simulink model "Vehicle_Model_14DOF"  (R2020a)
settings: Solver=ode23s  StartTime=0.0  StopTime=8  RelTol=1e-2  EnableMultiTasking=on
model workspace (MAT data in the model file):
  Csfl = 100
  Csfr = 100
  Csrl = 100
  Csrr = 100
  Hp = 0.35
  Ksfl = 100
  Ksfr = 100
  Ksrl = 100
  Ksrr = 100
undefined symbols (not defined in the file): sigbuilder_block
libraries: simulink_extras x6, simulink x1
(part 1 of 3)
settings Model: Creator=Admin  LastModifiedBy=Asser Roshdy
settings SolverCC: ZeroCrossControl=DisableAll
settings DataIOCC: ReturnWorkspaceOutputs=off
settings OptimizationCC: LifeSpan=inf
settings DebuggingCC: AllowSymbolicDim=off  StateNameClashWarn=warning  ArithmeticOperatorsInVariantConditions=warning
settings HardwareCC: ProdBitPerSizeT=32  ProdBitPerPtrDiffT=32  ProdWordSize=32  ProdHWDeviceType=Specified
settings SFSimCC: SimUseLocalCustomCode=off  CustomCodeUndefinedFunction=UseInterfaceOnly
settings RTWCC: RTWUseLocalCustomCode=off
settings CodeAppCC: StateflowObjectComments=on
settings SimscapeCC: SimscapeNormalizeSystem=off
settings ConfigurationSet: Description=SimMechanics 2G

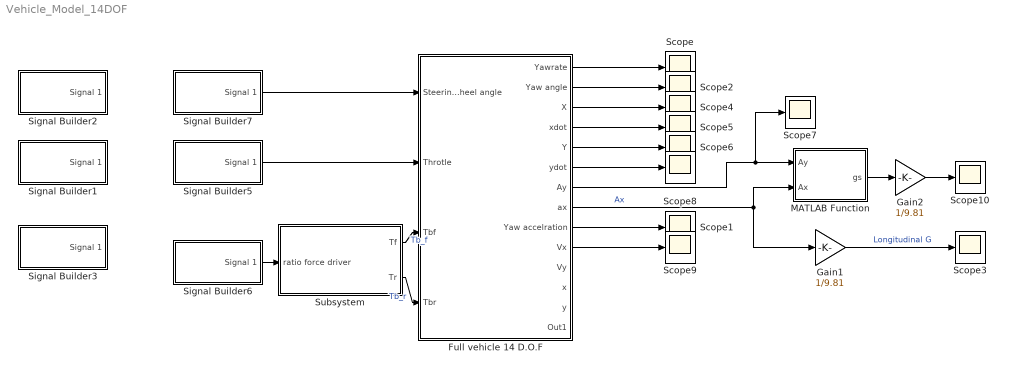
== system Vehicle_Model_14DOF ==
  "Full vehicle 14 D.O.F " : Subsystem  mask{P_A=0.75, Ms=240, Mufr=11.5, Mufl=11.5, Murr=13, Murl=13, wf=1.195, wr=1.180, b=0.753, a=0.826, H=0.314, Hr=0.060, Hp=0.096, Ip=38, Ir=146, Izz=125, Ksrr=16000, Ksrl=16000, Ksfr=21000, Ksfl=21000, Cdfr=781, Cdfl=781, Cdrr=944, Cdrl=944, Ktfr=120000, Ktfl=120000, Ktrr=120000, Ktrl=120000, Iwf=0.36, Iwr=0.36, Rw=0.260, R1=19.91, R2=13.86, R3=10.61, R4=8.535, Ro=1.18, Cd=0.91, Ar=1.2, Cl=2.1}
      mask prompts: P_A "Percentage Ackerman"; Ms "Sprung mass"; Mufr "Unsprung mass front right"; Mufl "Unsprung mass front left"; Murr "Unsprunf mass rear right"; Murl "Unsprunf mass rear left"; wf "Track width front"; wr "Track width rear"; b "C.G distance from the rear axle"; a "C.G distance from the front axle"; H "CG height"; Hr "Roll center height"; Hp "pitch center height"; Ip "Ixx"; Ir "Iyy"; Ksrr "Rear right susspension spring stiffness"; Ksrl "Rear left susspension spring stiffness"; Ksfr "Front right susspension spring stiffness"; Ksfl "Front left susspension spring stiffness"; Cdfr "Damping coefcient front right"; Cdfl "Damping coefcient front left"; Cdrr "Damping coefcient rear right"; Cdrl "Damping coefcient rear right"; Ktfr "Tire stiffness front right"; Ktfl "Tire stiffness front left"; Ktrr "Tire stiffness rear right"; Ktrl "Tire stiffness rear left"; Iwf "Tire inertia front"; Iwr "Tire inertia rear"; Rw "Tire rolling radius"; R1 "reduction 1"; R2 "reduction 2"; R3 "reduction 3"; R4 "reduction 4"; Ro "Air density"; Cd "Coefficient of drag"; Ar "Frontal area"; Cl "Coffiecient of downforce"
  Gain1 : Gain  Gain=1/9.81
  Gain2 : Gain  Gain=1/9.81
  MATLAB Function : MATLAB Function  TreatAsAtomicUnit=on
  Scope{,1..10} (11 alike) : Scope
  Signal Builder1 : Subsystem  Tag=STV Subsys  LoadFcn=sigbuilder_block('load');  StartFcn=sigbuilder_block('start');  StopFcn=sigbuilder_block('stop');  ClipboardFcn=sigbuilder_block('clipboard');  mask(Sigbuilder block){tuvar=[0:10]}
      mask help: Simulink:masks:SigbuilderBlock_MD
      mask init:
      | if ~strcmp(get_param(bdroot(gcbh),'SimulationStatus'),'stopped') tuvar = sigbuilder_block('maskInit'); end
      settings: CopyFcn=sigbuilder_block('copy');  DeleteFcn=sigbuilder_block('delete');  ModelCloseFcn=sigbuilder_block('modelClose');  PreSaveFcn=sigbuilder_block('preSave');  PauseFcn=sigbuilder_block('pause');  ContinueFcn=sigbuilder_block('continue');  NameChangeFcn=sigbuilder_block('namechange');  OpenFcn=sigbuilder_block('open',[84 117 1141.5 490.5 ]);  CloseFcn=sigbuilder_block('close');
      mask Display: plot(0, 0, 100, 100,[2, 2, 32, 32, 2], [68, 8, 8, 68, 68],[32, 2], [38, 38], [32, 19, 2],[53, 60, 44], [32, 17, 17, 2],[16, 16, 31, 31]);txt = getActiveGroup(gcbh);text(2, 100, txt,'verticalAlignment', 'top');
  Signal Builder2 : Subsystem  Tag=STV Subsys  LoadFcn=sigbuilder_block('load');  StartFcn=sigbuilder_block('start');  StopFcn=sigbuilder_block('stop');  ClipboardFcn=sigbuilder_block('clipboard');  mask(Sigbuilder block){tuvar=[0:10]}
      mask help: Simulink:masks:SigbuilderBlock_MD
      mask init:
      | if ~strcmp(get_param(bdroot(gcbh),'SimulationStatus'),'stopped') tuvar = sigbuilder_block('maskInit'); end
      settings: CopyFcn=sigbuilder_block('copy');  DeleteFcn=sigbuilder_block('delete');  ModelCloseFcn=sigbuilder_block('modelClose');  PreSaveFcn=sigbuilder_block('preSave');  PauseFcn=sigbuilder_block('pause');  ContinueFcn=sigbuilder_block('continue');  NameChangeFcn=sigbuilder_block('namechange');  OpenFcn=sigbuilder_block('open',[6 30 1428 681.75 ]);  CloseFcn=sigbuilder_block('close');
      mask Display: plot(0, 0, 100, 100,[2, 2, 32, 32, 2], [68, 8, 8, 68, 68],[32, 2], [38, 38], [32, 19, 2],[53, 60, 44], [32, 17, 17, 2],[16, 16, 31, 31]);txt = getActiveGroup(gcbh);text(2, 100, txt,'verticalAlignment', 'top');
  Signal Builder3 : Subsystem  Tag=STV Subsys  LoadFcn=sigbuilder_block('load');  StartFcn=sigbuilder_block('start');  StopFcn=sigbuilder_block('stop');  ClipboardFcn=sigbuilder_block('clipboard');  mask(Sigbuilder block){tuvar=[0:10]}
      mask help: Simulink:masks:SigbuilderBlock_MD
      mask init:
      | if ~strcmp(get_param(bdroot(gcbh),'SimulationStatus'),'stopped') tuvar = sigbuilder_block('maskInit'); end
      settings: CopyFcn=sigbuilder_block('copy');  DeleteFcn=sigbuilder_block('delete');  ModelCloseFcn=sigbuilder_block('modelClose');  PreSaveFcn=sigbuilder_block('preSave');  PauseFcn=sigbuilder_block('pause');  ContinueFcn=sigbuilder_block('continue');  NameChangeFcn=sigbuilder_block('namechange');  OpenFcn=sigbuilder_block('open',[20.25 37.5 1030.5 470.25 ]);  CloseFcn=sigbuilder_block('close');
      mask Display: plot(0, 0, 100, 100,[2, 2, 32, 32, 2], [68, 8, 8, 68, 68],[32, 2], [38, 38], [32, 19, 2],[53, 60, 44], [32, 17, 17, 2],[16, 16, 31, 31]);txt = getActiveGroup(gcbh);text(2, 100, txt,'verticalAlignment', 'top');
  Signal Builder5 : Subsystem  Tag=STV Subsys  LoadFcn=sigbuilder_block('load');  StartFcn=sigbuilder_block('start');  StopFcn=sigbuilder_block('stop');  ClipboardFcn=sigbuilder_block('clipboard');  mask(Sigbuilder block){tuvar=[0:10]}
      mask help: Simulink:masks:SigbuilderBlock_MD
      mask init:
      | if ~strcmp(get_param(bdroot(gcbh),'SimulationStatus'),'stopped') tuvar = sigbuilder_block('maskInit'); end
      settings: CopyFcn=sigbuilder_block('copy');  DeleteFcn=sigbuilder_block('delete');  ModelCloseFcn=sigbuilder_block('modelClose');  PreSaveFcn=sigbuilder_block('preSave');  PauseFcn=sigbuilder_block('pause');  ContinueFcn=sigbuilder_block('continue');  NameChangeFcn=sigbuilder_block('namechange');  OpenFcn=sigbuilder_block('open',[5.4 81 1141.2 421.8 ]);  CloseFcn=sigbuilder_block('close');
      mask Display: plot(0, 0, 100, 100,[2, 2, 32, 32, 2], [68, 8, 8, 68, 68],[32, 2], [38, 38], [32, 19, 2],[53, 60, 44], [32, 17, 17, 2],[16, 16, 31, 31]);txt = getActiveGroup(gcbh);text(2, 100, txt,'verticalAlignment', 'top');
  Signal Builder6 : Subsystem  Tag=STV Subsys  LoadFcn=sigbuilder_block('load');  StartFcn=sigbuilder_block('start');  StopFcn=sigbuilder_block('stop');  ClipboardFcn=sigbuilder_block('clipboard');  mask(Sigbuilder block){tuvar=[0:10]}
      mask help: Simulink:masks:SigbuilderBlock_MD
      mask init:
      | if ~strcmp(get_param(bdroot(gcbh),'SimulationStatus'),'stopped') tuvar = sigbuilder_block('maskInit'); end
      settings: CopyFcn=sigbuilder_block('copy');  DeleteFcn=sigbuilder_block('delete');  ModelCloseFcn=sigbuilder_block('modelClose');  PreSaveFcn=sigbuilder_block('preSave');  PauseFcn=sigbuilder_block('pause');  ContinueFcn=sigbuilder_block('continue');  NameChangeFcn=sigbuilder_block('namechange');  OpenFcn=sigbuilder_block('open',[5.4 173.4 1141.2 375.6 ]);  CloseFcn=sigbuilder_block('close');
      mask Display: plot(0, 0, 100, 100,[2, 2, 32, 32, 2], [68, 8, 8, 68, 68],[32, 2], [38, 38], [32, 19, 2],[53, 60, 44], [32, 17, 17, 2],[16, 16, 31, 31]);txt = getActiveGroup(gcbh);text(2, 100, txt,'verticalAlignment', 'top');
  Signal Builder7 : Subsystem  Tag=STV Subsys  LoadFcn=sigbuilder_block('load');  StartFcn=sigbuilder_block('start');  StopFcn=sigbuilder_block('stop');  ClipboardFcn=sigbuilder_block('clipboard');  mask(Sigbuilder block){tuvar=[0:10]}
      mask help: Simulink:masks:SigbuilderBlock_MD
      mask init:
      | if ~strcmp(get_param(bdroot(gcbh),'SimulationStatus'),'stopped') tuvar = sigbuilder_block('maskInit'); end
      settings: CopyFcn=sigbuilder_block('copy');  DeleteFcn=sigbuilder_block('delete');  ModelCloseFcn=sigbuilder_block('modelClose');  PreSaveFcn=sigbuilder_block('preSave');  PauseFcn=sigbuilder_block('pause');  ContinueFcn=sigbuilder_block('continue');  NameChangeFcn=sigbuilder_block('namechange');  OpenFcn=sigbuilder_block('open',[158.4 96.6 779.4 333.6 ]);  CloseFcn=sigbuilder_block('close');
      mask Display: plot(0, 0, 100, 100,[2, 2, 32, 32, 2], [68, 8, 8, 68, 68],[32, 2], [38, 38], [32, 19, 2],[53, 60, 44], [32, 17, 17, 2],[16, 16, 31, 31]);txt = getActiveGroup(gcbh);text(2, 100, txt,'verticalAlignment', 'top');
  Subsystem : Subsystem  mask{Fd=300, PR=3.5, a=75, b=25, Amf=403, Amr=483, Asf=793*2, Asr=509*2, rb=110, Mb=0.55}
      mask prompts: Fd "force driver"; PR "pedal ratio"; a "% brake bias front"; b "% brake bias rear"; Amf "Area master cylinder front"; Amr "Area master cylinder rear"; Asf "Area caliper front"; Asr "Area caliper rear"; rb "effective rotor radius"; Mb "coefficient of friction between the pad and the disc"
  wires:
  "Full vehicle 14 D.O.F "/2(Yaw angle) -> Scope2/1
  "Full vehicle 14 D.O.F "/3(X) -> Scope4/1
  "Full vehicle 14 D.O.F "/4(xdot) -> Scope5/1
  "Full vehicle 14 D.O.F "/6(ydot) -> Scope8/1
  "Full vehicle 14 D.O.F "/8(ax) -> Gain1/1, MATLAB Function/2(Ax)  "Ax"
  "Full vehicle 14 D.O.F "/7(Ay) -> Scope7/1, MATLAB Function/1(Ay)
  "Full vehicle 14 D.O.F "/5(Y) -> Scope6/1
  "Full vehicle 14 D.O.F "/9("Yaw accelration ") -> Scope1/1
  Subsystem/1(Tf) -> "Full vehicle 14 D.O.F "/3("Tbf ")  "Tb_f"
  Subsystem/2(Tr) -> "Full vehicle 14 D.O.F "/4("Tbr ")  "Tb_r"
  "Full vehicle 14 D.O.F "/10(Vx) -> Scope9/1
  MATLAB Function/1(gs) -> Gain2/1
  Gain2/1 -> Scope10/1
  "Full vehicle 14 D.O.F "/1(Yawrate) -> Scope/1
  Signal Builder7/1(Signal 1) -> "Full vehicle 14 D.O.F "/1("Steering wheel angle ")
  Signal Builder5/1(Signal 1) -> "Full vehicle 14 D.O.F "/2("Throtle ")
  Signal Builder6/1(Signal 1) -> Subsystem/1(ratio force driver)
  Gain1/1 -> Scope3/1  "Longitudinal G"

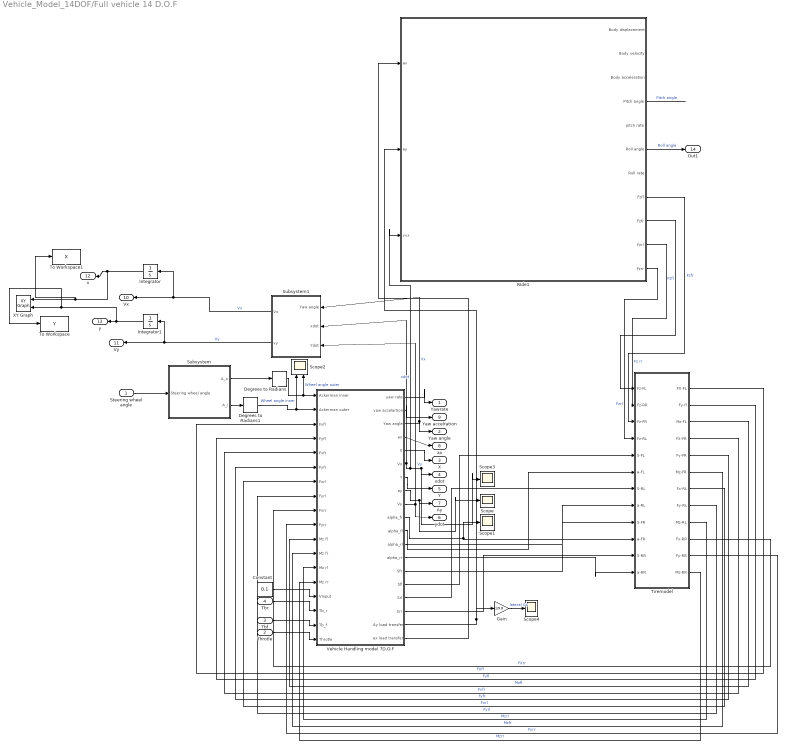
== system Vehicle_Model_14DOF/Full vehicle 14 D.O.F  ==
  "Steering wheel angle " : Inport
  "Throtle " : Inport  Port=2
  "Tbf " : Inport  Port=3
  "Tbr " : Inport  Port=4
  Constant : Constant  Value=0.1
  Degrees to Radians : simulink_extras/Transformations/Degrees to Radians
  Degrees to Radians1 : simulink_extras/Transformations/Degrees to Radians
  Gain : Gain  Gain=1/9.8
  Integrator : Integrator
  Integrator1 : Integrator
  RIde1 : Subsystem
  Scope{,1,3..4} (4 alike) : Scope
  Scope2 : Scope  NumInputPorts=2
  Subsystem : Subsystem
  Subsystem1 : Subsystem
  Tiremodel : Subsystem
  To Workspace : ToWorkspace  VariableName=Y  SaveFormat=Timeseries  SampleTime=-1
  To Workspace1 : ToWorkspace  VariableName=X  SaveFormat=Timeseries  SampleTime=-1
  "Vehicle Handling model 7D.O.F " : Subsystem
  XY Graph : simulink/Sinks/XY Graph  xmin=-200  xmax=200  ymin=-200  ymax=200  st=-1
  Yawrate : Outport  VectorParamsAs1DForOutWhenUnconnected=off
  Yaw angle : Outport  Port=2  VectorParamsAs1DForOutWhenUnconnected=off
  X : Outport  Port=3  VectorParamsAs1DForOutWhenUnconnected=off
  xdot : Outport  Port=4  VectorParamsAs1DForOutWhenUnconnected=off
  Y : Outport  Port=5  VectorParamsAs1DForOutWhenUnconnected=off
  ydot : Outport  Port=6  VectorParamsAs1DForOutWhenUnconnected=off
  Ay : Outport  Port=7  VectorParamsAs1DForOutWhenUnconnected=off
  ax : Outport  Port=8  VectorParamsAs1DForOutWhenUnconnected=off
  "Yaw accelration " : Outport  Port=9  VectorParamsAs1DForOutWhenUnconnected=off
  Vx : Outport  Port=10  VectorParamsAs1DForOutWhenUnconnected=off
  Vy : Outport  Port=11  VectorParamsAs1DForOutWhenUnconnected=off
  x : Outport  Port=12  VectorParamsAs1DForOutWhenUnconnected=off
  y : Outport  Port=13  VectorParamsAs1DForOutWhenUnconnected=off
  Out1 : Outport  Port=14  VectorParamsAs1DForOutWhenUnconnected=off
  wires:
  Constant/1 -> "Vehicle Handling model 7D.O.F "/15("Vinput ")
  "Vehicle Handling model 7D.O.F "/1(yaw rate) -> Yawrate/1
  "Vehicle Handling model 7D.O.F "/5(X) -> X/1
  "Vehicle Handling model 7D.O.F "/4(ax) -> ax/1
  "Vehicle Handling model 7D.O.F "/3(Yaw angle) -> Subsystem1/1(Yaw angle), Yaw angle/1  "Vx"
  "Vehicle Handling model 7D.O.F "/6(Vx) -> Subsystem1/2(xdot), RIde1/3(vvx), Scope3/1, xdot/1  "xdot"
  "Vehicle Handling model 7D.O.F "/7(Y) -> Y/1
  "Vehicle Handling model 7D.O.F "/8(ay) -> Ay/1, Scope/1
  "Vehicle Handling model 7D.O.F "/9(Vy) -> ydot/1, Subsystem1/3(Ydot)  "Vy"
  "Vehicle Handling model 7D.O.F "/2("yaw accelartion ") -> "Yaw accelration "/1
  "Vehicle Handling model 7D.O.F "/14(Sfr) -> Tiremodel/9(S-FR)
  "Vehicle Handling model 7D.O.F "/15(Sfl) -> Tiremodel/5(S-FL)
  "Vehicle Handling model 7D.O.F "/16(Srl) -> Tiremodel/7(S-RL)
  "Vehicle Handling model 7D.O.F "/17(Srr) -> Tiremodel/11(S-RR)
  "Vehicle Handling model 7D.O.F "/10(alpha_fr) -> Tiremodel/10(a-FR), Scope1/1
  "Vehicle Handling model 7D.O.F "/11(alpha_fl) -> Tiremodel/6(a-FL)
  "Vehicle Handling model 7D.O.F "/12(alpha_rl) -> Tiremodel/8(a-RL)
  "Vehicle Handling model 7D.O.F "/13(alpha_rr) -> Tiremodel/12(a-RR)
  Tiremodel/1(FX-FL) -> "Vehicle Handling model 7D.O.F "/3(Fxfl)  "FXfl"
  Tiremodel/2(Fy-fl) -> "Vehicle Handling model 7D.O.F "/4("Fyfl ")  "Fyfl"
  Tiremodel/3(Mz-FL) -> "Vehicle Handling model 7D.O.F "/11(Mz fl)  "Mzfl"
  Tiremodel/4(FX-FR) -> "Vehicle Handling model 7D.O.F "/5(Fxfr)  "Fxfr"
  Tiremodel/5(Fy-FR) -> "Vehicle Handling model 7D.O.F "/6(Fyfr)  "fyfr"
  Tiremodel/7(Fx-RL) -> "Vehicle Handling model 7D.O.F "/7(Fxrl)  "Fxrl"
  Tiremodel/8(Fy-RL) -> "Vehicle Handling model 7D.O.F "/8(Fyrl)  "Fyrl"
  Tiremodel/9(Mz-RL) -> "Vehicle Handling model 7D.O.F "/13(Mz rl)  "Mzrl"
  Tiremodel/10(Fx-RR) -> "Vehicle Handling model 7D.O.F "/9(Fxrr)  "FXrr"
  Tiremodel/6(Mz-FR) -> "Vehicle Handling model 7D.O.F "/12(Mz fr)  "Mzfr"
  Tiremodel/11(Fy-RR) -> "Vehicle Handling model 7D.O.F "/10(Fyrr)  "Fyrr"
  Tiremodel/12(Mz-RR) -> "Vehicle Handling model 7D.O.F "/14(Mz rr)  "Mzrr"
  "Throtle "/1 -> "Vehicle Handling model 7D.O.F "/18(Throtle)
  "Tbr "/1 -> "Vehicle Handling model 7D.O.F "/16(Tb_r)
  "Tbf "/1 -> "Vehicle Handling model 7D.O.F "/17(Tb_f)
  "Steering wheel angle "/1 -> Subsystem/1("Steering wheel angle ")
  Subsystem/2("A_i ") -> Degrees to Radians1/1
  Degrees to Radians1/1 -> Scope2/1, "Vehicle Handling model 7D.O.F "/2(Ackerman outer)  "Wheel angle inner"
  Degrees to Radians/1 -> "Vehicle Handling model 7D.O.F "/1(Ackerman inner), Scope2/2  "Wheel angle outer"
  Subsystem1/1(Vx) -> Integrator/1, Vx/1  "Vx"
  Subsystem1/2(vy) -> Integrator1/1, Vy/1  "Vy"
  Integrator/1 -> To Workspace1/1, XY Graph/1, x/1
  Integrator1/1 -> To Workspace/1, XY Graph/2, y/1
  Subsystem/1(A_o) -> Degrees to Radians/1
  RIde1/4(Pitch angle) -> ?  "Pitch angle"
  RIde1/11(Fzrr) -> Tiremodel/4(Fz-RL)  "Fzrl"
  RIde1/10(Fzrl) -> Tiremodel/2(Fz-RR)  "Fz rr"
  RIde1/9(Fzfr) -> Tiremodel/1(Fz-FL)  "Fzfl"
  RIde1/8(Fzfl) -> Tiremodel/3(Fz-FR)  "Fzfr"
  RIde1/6(Roll angle) -> Out1/1  "Roll angle"
  "Vehicle Handling model 7D.O.F "/19(ax load transfer) -> RIde1/1(ax)
  "Vehicle Handling model 7D.O.F "/18(Ay load transfer) -> Gain/1, RIde1/2(ay)
  Gain/1 -> Scope4/1  "lateral Gs"

== system Vehicle_Model_14DOF/Signal Builder1 ==
  Demux : Demux  Tag=STV Demux  Outputs=1
      settings: DisplayOption=none
  FromWs : FromWorkspace  Tag=STV FromWs  VariableName=tuvar
      SigBuilderData=|
      | common.afterFinalStr = 'Extrapolate'
      | common.sampleTime = 0
      | dataSet.timeRange = [0 24]
      | dataSet.name = 'Group 1'
      | sbobj.Groups.Name = 'Group 1'
      | sbobj.Groups.Signals.Name = 'Signal 1'
      | sbobj.Groups.Signals.XData = [0 2.95 3.5 3.95 4.35 4.8 4.95 5.15 7.15 7.25 8.15 8.25 8.45 8.85 8.95 9.55 10.05 11.35 11.45 12.15 12.25 12.35 12.4 12.45 12.55 13.55 14.2 15.15 15.7 16.2 17 17.55 18.05 19.05 19.5 20.15 20.9 21.3 24]
      | sbobj.Groups.Signals.YData = [1 1 0.4 0.55 0.4 0.5 0.5 0 0 1 1 0.75 0.5 0.5 0.2 0.2 1 1 0 0 0.1 0.25 0.25 0 0 0 0 0 0 0 0 0 0 0 0 0 0 0 0]
      | sbobj.Groups.TimeRange = [0 24]
  Signal 1 : Outport  Tag=STV Outport  VectorParamsAs1DForOutWhenUnconnected=off
  wires:
  Demux/1 -> Signal 1/1
  FromWs/1 -> Demux/1

== system Vehicle_Model_14DOF/Signal Builder2 ==
  Demux : Demux  Tag=STV Demux  Outputs=1
      settings: DisplayOption=none
  FromWs : FromWorkspace  Tag=STV FromWs  VariableName=tuvar
      SigBuilderData=|
      | common.afterFinalStr = 'Extrapolate'
      | common.sampleTime = 0
      | dataSet.timeRange = [0 24]
      | dataSet.name = 'Group 1'
      | sbobj.Groups.Name = 'Group 1'
      | sbobj.Groups.Signals.Name = 'Signal 1'
      | sbobj.Groups.Signals.XData = [0 3 3.2 3.5 3.65 3.8 3.95 4 4.1 4.15 4.25 4.3 4.6 4.85 5 5.1 5.45 5.5 5.6 5.65 5.7 5.85 5.9 5.95 6.1 6.3 6.4 6.45 6.6 7.15 7.45 8.55 8.7 8.75 8.85 9 9.1 9.15 9.25 9.3 9.4 9.75 9.95 10.05 10.1 10.15 10.25 11.95 12.05 12.25 12.35 12.45 12.55 12.65 12.7 12.8 12.85 24]
      | sbobj.Groups.Signals.YData = [0 0 50 50 0 -50 -50 0 50 50 0 -10 -10 -10 0 10 10 0 -30 -30 0 0 30 30 0 0 40 80 90 90 0 0 -50 -50 0 0 30 30 60 60 40 50 50 0 -10 -25 0 0 -25 -25 -35 -52 -70 -70 -25 -25 0 0]
      | sbobj.Groups.TimeRange = [0 24]
  Signal 1 : Outport  Tag=STV Outport  VectorParamsAs1DForOutWhenUnconnected=off
  wires:
  Demux/1 -> Signal 1/1
  FromWs/1 -> Demux/1

== system Vehicle_Model_14DOF/Signal Builder3 ==
  Demux : Demux  Tag=STV Demux  Outputs=1
      settings: DisplayOption=none
  FromWs : FromWorkspace  Tag=STV FromWs  VariableName=tuvar
      SigBuilderData=|
      | common.afterFinalStr = 'Extrapolate'
      | common.sampleTime = 0
      | dataSet.timeRange = [0 24]
      | dataSet.name = 'Group 1'
      | sbobj.Groups.Name = 'Group 1'
      | sbobj.Groups.Signals.Name = 'Signal 1'
      | sbobj.Groups.Signals.XData = [0 5.05 5.1 5.2 5.35 5.5 5.6 5.7 5.85 6.3 6.35 6.55 6.65 11.35 11.5 12 12.1 12.45 12.65 12.7 14.6 15 16 17.35 24]
      | sbobj.Groups.Signals.YData = [0 0 0.3 0.99 0.99 0.25 0.5 0.75 0.75 0.65 0.1 0.3 0 0 0.99 0.99 0 0.99 0.99 0 0 0 0 0 0.00475]
      | sbobj.Groups.TimeRange = [0 24]
  Signal 1 : Outport  Tag=STV Outport  VectorParamsAs1DForOutWhenUnconnected=off
  wires:
  Demux/1 -> Signal 1/1
  FromWs/1 -> Demux/1

== system Vehicle_Model_14DOF/Signal Builder5 ==
  Demux : Demux  Tag=STV Demux  Outputs=1
      settings: DisplayOption=none
  FromWs : FromWorkspace  Tag=STV FromWs  VariableName=tuvar
      SigBuilderData=|
      | common.afterFinalStr = 'Extrapolate'
      | common.sampleTime = 0
      | dataSet.timeRange = [0 24]
      | dataSet.name = 'Group 1'
      | sbobj.Groups.Name = 'Group 1'
      | sbobj.Groups.Signals.Name = 'Signal 1'
      | sbobj.Groups.Signals.XData = [0 2 2 24]
      | sbobj.Groups.Signals.YData = [0.995 0.995 0.2 0.2]
      | sbobj.Groups.TimeRange = [0 24]
  Signal 1 : Outport  Tag=STV Outport  VectorParamsAs1DForOutWhenUnconnected=off
  wires:
  Demux/1 -> Signal 1/1
  FromWs/1 -> Demux/1

== system Vehicle_Model_14DOF/Signal Builder6 ==
  Demux : Demux  Tag=STV Demux  Outputs=1
      settings: DisplayOption=none
  FromWs : FromWorkspace  Tag=STV FromWs  VariableName=tuvar
      SigBuilderData=|
      | common.afterFinalStr = 'Extrapolate'
      | common.sampleTime = 0
      | dataSet.timeRange = [0 24]
      | dataSet.name = 'Group 1'
      | sbobj.Groups.Name = 'Group 1'
      | sbobj.Groups.Signals.Name = 'Signal 1'
      | sbobj.Groups.Signals.XData = [0 2 2 3 3 24]
      | sbobj.Groups.Signals.YData = [0 0 0.195 0.195 0 0]
      | sbobj.Groups.TimeRange = [0 24]
  Signal 1 : Outport  Tag=STV Outport  VectorParamsAs1DForOutWhenUnconnected=off
  wires:
  Demux/1 -> Signal 1/1
  FromWs/1 -> Demux/1

== system Vehicle_Model_14DOF/Signal Builder7 ==
  Demux : Demux  Tag=STV Demux  Outputs=1
      settings: DisplayOption=none
  FromWs : FromWorkspace  Tag=STV FromWs  VariableName=tuvar
      SigBuilderData=|
      | common.afterFinalStr = 'Extrapolate'
      | common.sampleTime = 0
      | dataSet.timeRange = [0 24]
      | dataSet.name = 'Group 1'
      | sbobj.Groups.Name = 'Group 1'
      | sbobj.Groups.Signals.Name = 'Signal 1'
      | sbobj.Groups.Signals.XData = [0 2 2.1 24]
      | sbobj.Groups.Signals.YData = [0 0 105 105]
      | sbobj.Groups.TimeRange = [0 24]
  Signal 1 : Outport  Tag=STV Outport  VectorParamsAs1DForOutWhenUnconnected=off
  wires:
  Demux/1 -> Signal 1/1
  FromWs/1 -> Demux/1

== system Vehicle_Model_14DOF/Subsystem ==
  ratio force driver : Inport
  Gain : Gain  Gain=1/1000
  Gain1 : Gain  Gain=1/1000
  Subsystem : Subsystem
  Subsystem1 : Subsystem
  Subsystem2 : Subsystem
  Subsystem3 : Subsystem
  Subsystem4 : Subsystem
  Subsystem5 : Subsystem
  Subsystem6 : Subsystem
  Subsystem7 : Subsystem
  Subsystem8 : Subsystem
  Tf : Outport  VectorParamsAs1DForOutWhenUnconnected=off
  Tr : Outport  Port=2  VectorParamsAs1DForOutWhenUnconnected=off
  wires:
  Gain1/1 -> Tr/1
  Gain/1 -> Tf/1
  ratio force driver/1 -> Subsystem8/1(%Fd)
  Subsystem8/1(Fb) -> Subsystem7/1(Fb), Subsystem6/1(Fb)
  Subsystem7/1(Fr) -> Subsystem3/1(Fr)
  Subsystem6/1(Ff) -> Subsystem/1(Ff)
  Subsystem5/1(Tr) -> Gain1/1
  Subsystem2/1(Tf) -> Gain/1
  Subsystem4/1(Fcr) -> Subsystem5/1(Fcr)
  Subsystem3/1(Pr) -> Subsystem4/1(Pr)
  Subsystem1/1(Fcf) -> Subsystem2/1(Fcf)
  Subsystem/1(Pf) -> Subsystem1/1(Pf)

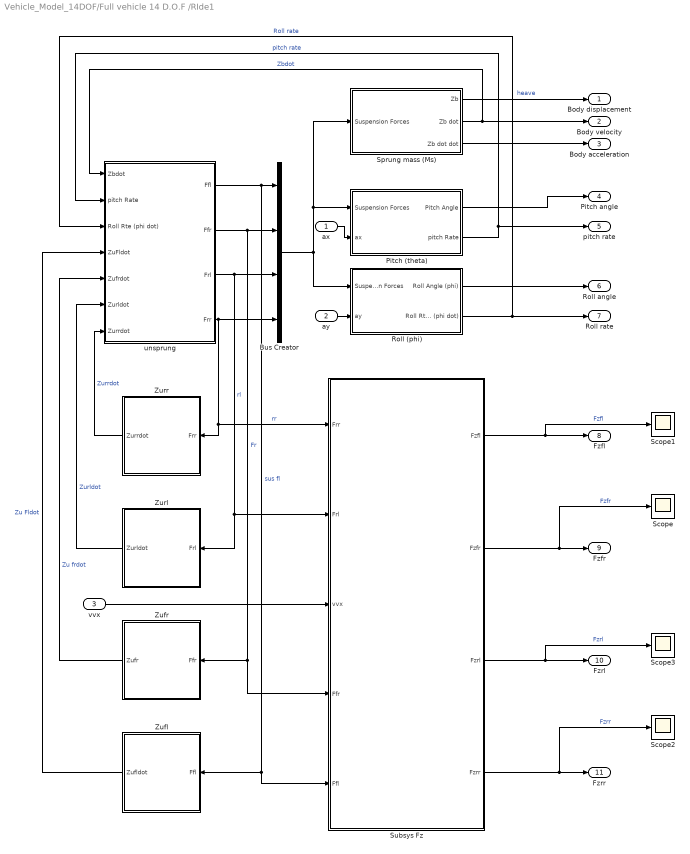
== system Vehicle_Model_14DOF/Full vehicle 14 D.O.F /RIde1 ==
  ax : Inport
  ay : Inport  Port=2
  vvx : Inport  Port=3
  Bus Creator : BusCreator  Inputs=4
  Pitch (theta) : Subsystem
  Roll (phi) : Subsystem
  Scope{,1..3} (4 alike) : Scope
  Sprung mass (Ms) : Subsystem
  Subsys Fz : Subsystem
  Zufl : Subsystem
  Zufr : Subsystem
  Zurl : Subsystem
  Zurr : Subsystem
  unsprung : Subsystem
  Body displacement : Outport  VectorParamsAs1DForOutWhenUnconnected=off
  Body velocity : Outport  Port=2  VectorParamsAs1DForOutWhenUnconnected=off
  Body acceleration : Outport  Port=3  VectorParamsAs1DForOutWhenUnconnected=off
  Pitch angle : Outport  Port=4  VectorParamsAs1DForOutWhenUnconnected=off
  pitch rate : Outport  Port=5  VectorParamsAs1DForOutWhenUnconnected=off
  Roll angle : Outport  Port=6  VectorParamsAs1DForOutWhenUnconnected=off
  Roll rate : Outport  Port=7  VectorParamsAs1DForOutWhenUnconnected=off
  Fzfl : Outport  Port=8  VectorParamsAs1DForOutWhenUnconnected=off
  Fzfr : Outport  Port=9  VectorParamsAs1DForOutWhenUnconnected=off
  Fzrl : Outport  Port=10  VectorParamsAs1DForOutWhenUnconnected=off
  Fzrr : Outport  Port=11  VectorParamsAs1DForOutWhenUnconnected=off
  wires:
  Zurr/1(Zurrdot) -> unsprung/7(Zurrdot)  "Zurrdot"
  unsprung/4(Frr) -> Zurr/1(Frr), Subsys Fz/1(Frr), Bus Creator/4  "rr"
  unsprung/2(Ffr) -> Bus Creator/2, Zufr/1(Ffr), Subsys Fz/4(Ffr)  "Fr"
  Bus Creator/1 -> Sprung mass (Ms)/1(Suspension Forces), Pitch (theta)/1(Suspension Forces), Roll (phi)/1(Suspension Forces)
  Roll (phi)/1(Roll Angle (phi)) -> Roll angle/1
  unsprung/3(Frl) -> Zurl/1(Frl), Subsys Fz/2(Frl), Bus Creator/3  "rl"
  Roll (phi)/2(Roll Rte (phi dot)) -> Roll rate/1, unsprung/3(Roll Rte (phi dot))  "Roll rate"
  unsprung/1(Ffl) -> Zufl/1(Ffl), Subsys Fz/5(Ffl), Bus Creator/1  "sus fl"
  Sprung mass (Ms)/2(Zb dot) -> Body velocity/1, unsprung/1(Zbdot)  "Zbdot"
  Pitch (theta)/1(Pitch Angle) -> Pitch angle/1
  Sprung mass (Ms)/1(Zb) -> Body displacement/1  "heave"
  Zufr/1(Zufr) -> unsprung/5(Zufrdot)  "Zu frdot"
  Pitch (theta)/2(pitch Rate) -> pitch rate/1, unsprung/2(pitch Rate)  "pitch rate"
  Zurl/1(Zurldot) -> unsprung/6(Zurldot)  "Zurldot"
  Subsys Fz/2(Fzfr) -> Scope/1, Fzfr/1  "Fzfr"
  Sprung mass (Ms)/3(Zb dot dot) -> Body acceleration/1
  Zufl/1(Zufldot) -> unsprung/4(ZuFldot)  "Zu Fldot"
  ax/1 -> Pitch (theta)/2(ax)
  ay/1 -> Roll (phi)/2(ay)
  Subsys Fz/1(Fzfl) -> Scope1/1, Fzfl/1  "Fzfl"
  Subsys Fz/3(Fzrl) -> Scope3/1, Fzrl/1  "Fzrl"
  Subsys Fz/4(Fzrr) -> Scope2/1, Fzrr/1  "Fzrr"
  vvx/1 -> Subsys Fz/3(vvx)

== system Vehicle_Model_14DOF/Full vehicle 14 D.O.F /Subsystem ==
  "Steering wheel angle " : Inport
  Constant : Constant  Value=a
  Constant1 : Constant  Value=b
  Constant2 : Constant  Value=wf
  Constant3 : Constant  Value=P_A
  MATLAB Function : MATLAB Function  TreatAsAtomicUnit=on
  Steering ratio : Gain  Gain=1/6
  A_o : Outport  VectorParamsAs1DForOutWhenUnconnected=off
  "A_i " : Outport  Port=2  VectorParamsAs1DForOutWhenUnconnected=off
  wires:
  MATLAB Function/1(Ackerman_inner) -> "A_i "/1
  "Steering wheel angle "/1 -> Steering ratio/1
  Constant2/1 -> MATLAB Function/4(Wf)
  Steering ratio/1 -> MATLAB Function/1(Ackerman), A_o/1
  Constant/1 -> MATLAB Function/2(a)
  Constant1/1 -> MATLAB Function/3(b)
  Constant3/1 -> MATLAB Function/5(Percent)

== system Vehicle_Model_14DOF/Full vehicle 14 D.O.F /Subsystem1 ==
  Yaw angle : Inport
  xdot : Inport  Port=2
  Ydot : Inport  Port=3
  Add : Sum  Inputs=+-
  Add1 : Sum
  Cos : Trigonometry  Operator=cos
  Product{,1..3} (4 alike) : Product
  Sin : Trigonometry
  Vx : Outport  VectorParamsAs1DForOutWhenUnconnected=off
  vy : Outport  Port=2  VectorParamsAs1DForOutWhenUnconnected=off
  wires:
  xdot/1 -> Product2/1, Product/1
  Sin/1 -> Product2/2, Product1/2
  Cos/1 -> Product3/2, Product/2
  Yaw angle/1 -> Product3/1, Sin/1, Cos/1
  Product2/1 -> Add1/1
  Product/1 -> Add/1
  Product1/1 -> Add/2
  Product3/1 -> Add1/2
  Ydot/1 -> Product1/1
  Add/1 -> Vx/1
  Add1/1 -> vy/1

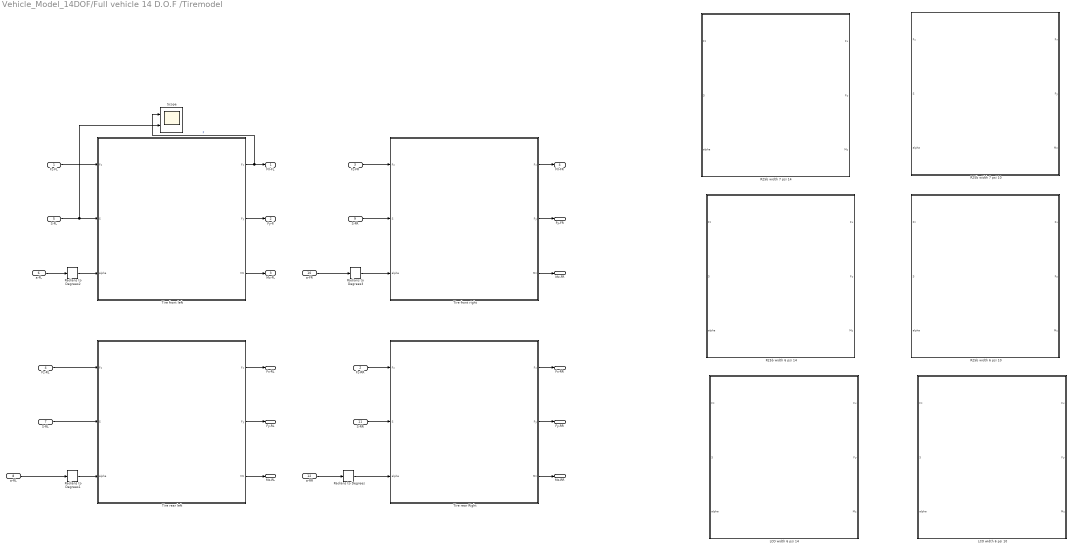
== system Vehicle_Model_14DOF/Full vehicle 14 D.O.F /Tiremodel ==
  Fz-FL : Inport
  Fz-RR : Inport  Port=2
  Fz-FR : Inport  Port=3
  Fz-RL : Inport  Port=4
  S-FL : Inport  Port=5
  a-FL : Inport  Port=6
  S-RL : Inport  Port=7
  a-RL : Inport  Port=8
  S-FR : Inport  Port=9
  a-FR : Inport  Port=10
  S-RR : Inport  Port=11
  a-RR : Inport  Port=12
  LCO width 6 psi 10 : Subsystem
  LCO width 6 psi 14 : Subsystem
  R25b width 6 psi 10 : Subsystem
  R25b width 6 psi 14 : Subsystem
  R25b width 7 psi 10 : Subsystem
  R25b width 7 psi 14 : Subsystem
  Radians to Degrees{,1..3} (4 alike) : simulink_extras/Transformations/Radians to Degrees
  Scope : Scope  NumInputPorts=2
  Tire front left : Subsystem
  Tire front right : Subsystem
  Tire rear Right : Subsystem
  Tire rear left : Subsystem
  FX-FL : Outport  VectorParamsAs1DForOutWhenUnconnected=off
  Fy-fl : Outport  Port=2  VectorParamsAs1DForOutWhenUnconnected=off
  Mz-FL : Outport  Port=3  VectorParamsAs1DForOutWhenUnconnected=off
  FX-FR : Outport  Port=4  VectorParamsAs1DForOutWhenUnconnected=off
  Fy-FR : Outport  Port=5  VectorParamsAs1DForOutWhenUnconnected=off
  Mz-FR : Outport  Port=6  VectorParamsAs1DForOutWhenUnconnected=off
  Fx-RL : Outport  Port=7  VectorParamsAs1DForOutWhenUnconnected=off
  Fy-RL : Outport  Port=8  VectorParamsAs1DForOutWhenUnconnected=off
  Mz-RL : Outport  Port=9  VectorParamsAs1DForOutWhenUnconnected=off
  Fx-RR : Outport  Port=10  VectorParamsAs1DForOutWhenUnconnected=off
  Fy-RR : Outport  Port=11  VectorParamsAs1DForOutWhenUnconnected=off
  Mz-RR : Outport  Port=12  VectorParamsAs1DForOutWhenUnconnected=off
  wires:
  Fz-FL/1 -> Tire front left/1(Fz)
  Fz-RR/1 -> Tire rear Right/1(Fz)
  S-FL/1 -> Scope/2, Tire front left/2(S)
  Fz-RL/1 -> Tire rear left/1(Fz)
  S-RL/1 -> Tire rear left/2(S)
  a-RL/1 -> Radians to Degrees1/1
  Fz-FR/1 -> Tire front right/1(Fz)
  S-FR/1 -> Tire front right/2(S)
  S-RR/1 -> Tire rear Right/2(S)
  Tire front left/1("Fx  ") -> Scope/1, FX-FL/1  "F"
  Tire front left/2(Fy) -> Fy-fl/1
  Tire front left/3(Mz) -> Mz-FL/1
  Tire front right/1("Fx  ") -> FX-FR/1
  Tire front right/2(Fy) -> Fy-FR/1
  Tire front right/3(Mz) -> Mz-FR/1
  Tire rear left/1("Fx  ") -> Fx-RL/1
  Tire rear left/2(Fy) -> Fy-RL/1
  Tire rear left/3(Mz) -> Mz-RL/1
  Tire rear Right/3(Mz) -> Mz-RR/1
  Tire rear Right/2(Fy) -> Fy-RR/1
  Tire rear Right/1("Fx  ") -> Fx-RR/1
  a-FL/1 -> Radians to Degrees2/1
  a-FR/1 -> Radians to Degrees3/1
  Radians to Degrees1/1 -> Tire rear left/3(alpha)
  a-RR/1 -> Radians to Degrees/1
  Radians to Degrees/1 -> Tire rear Right/3(alpha)
  Radians to Degrees2/1 -> Tire front left/3(alpha)
  Radians to Degrees3/1 -> Tire front right/3(alpha)

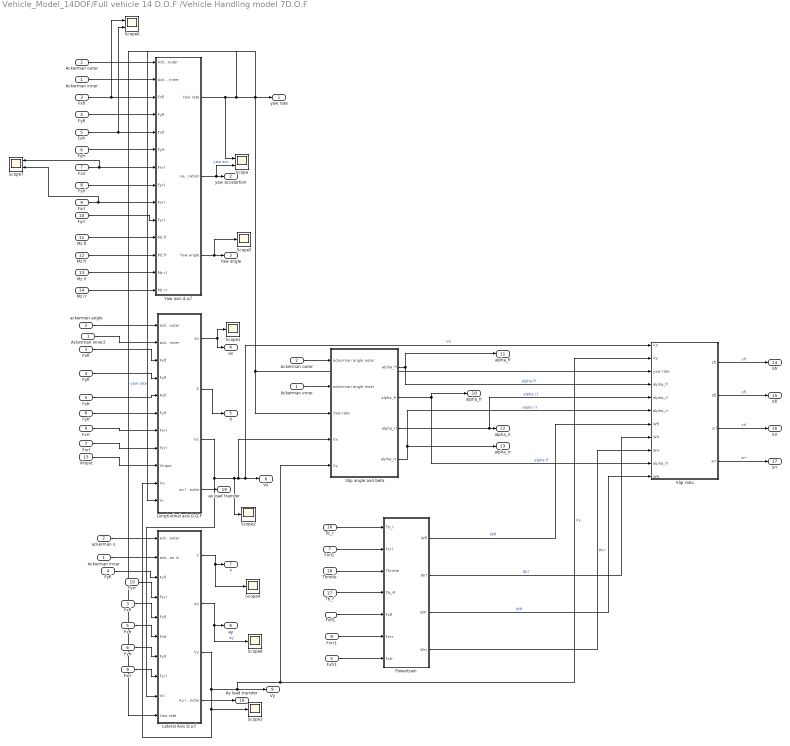
== system Vehicle_Model_14DOF/Full vehicle 14 D.O.F /Vehicle Handling model 7D.O.F  ==
  Ackerman inner : Inport
  Ackerman outer : Inport  Port=2
  Fxfl : Inport  Port=3
  "Fyfl " : Inport  Port=4
  Fxfr : Inport  Port=5
  Fyfr : Inport  Port=6
  Fxrl : Inport  Port=7
  Fyrl : Inport  Port=8
  Fxrr : Inport  Port=9
  Fyrr : Inport  Port=10
  Mz fl : Inport  Port=11
  Mz fr : Inport  Port=12
  Mz rl : Inport  Port=13
  Mz rr : Inport  Port=14
  "Vinput " : Inport  Port=15
  Tb_r : Inport  Port=16
  Tb_f : Inport  Port=17
  Throtle : Inport  Port=18
  "Ackerman inner " : InportShadow
  "Ackerman inner " : InportShadow
  Ackerman inner2 : InportShadow
  "Ackerman outer " : InportShadow  Port=2
  "Fxfl " : InportShadow  Port=3
  "Fxfl " : InportShadow  Port=3
  Fxfl1 : InportShadow  Port=3
  "Fxfr " : InportShadow  Port=5
  "Fxfr " : InportShadow  Port=5
  Fxfr1 : InportShadow  Port=5
  "Fxrl " : InportShadow  Port=7
  Fxrl1 : InportShadow  Port=7
  "Fxrr " : InportShadow  Port=9
  "Fxrr " : InportShadow  Port=9
  Fxrr1 : InportShadow  Port=9
  Fyfl : InportShadow  Port=4
  "Fyfl " : InportShadow  Port=4
  "Fyfr " : InportShadow  Port=6
  "Fyfr " : InportShadow  Port=6
  "Fyrr    " : InportShadow  Port=10
  "Lateral Axis D.o.f " : Subsystem
  "Longtudinal axis D.O.F " : Subsystem
  "Powertrain " : Subsystem
  Scope : Scope  NumInputPorts=2
  Scope{1..5,8} (6 alike) : Scope
  Scope6 : Scope  NumInputPorts=2
  Scope7 : Scope  NumInputPorts=2
  "Slip angle and beta " : Subsystem
  "Slip ratio " : Subsystem
  "Yaw axis d,o,f " : Subsystem
  "ackerman angle " : InportShadow  Port=2
  "ackerman o " : InportShadow  Port=2
  yaw rate : Outport  VectorParamsAs1DForOutWhenUnconnected=off
  "yaw accelartion " : Outport  Port=2  VectorParamsAs1DForOutWhenUnconnected=off
  Yaw angle : Outport  Port=3  VectorParamsAs1DForOutWhenUnconnected=off
  ax : Outport  Port=4  VectorParamsAs1DForOutWhenUnconnected=off
  X : Outport  Port=5  VectorParamsAs1DForOutWhenUnconnected=off
  Vx : Outport  Port=6  VectorParamsAs1DForOutWhenUnconnected=off
  Y : Outport  Port=7  VectorParamsAs1DForOutWhenUnconnected=off
  ay : Outport  Port=8  VectorParamsAs1DForOutWhenUnconnected=off
  Vy : Outport  Port=9  VectorParamsAs1DForOutWhenUnconnected=off
  alpha_fr : Outport  Port=10  VectorParamsAs1DForOutWhenUnconnected=off
  alpha_fl : Outport  Port=11  VectorParamsAs1DForOutWhenUnconnected=off
  alpha_rl : Outport  Port=12  VectorParamsAs1DForOutWhenUnconnected=off
  alpha_rr : Outport  Port=13  VectorParamsAs1DForOutWhenUnconnected=off
  Sfr : Outport  Port=14  VectorParamsAs1DForOutWhenUnconnected=off
  Sfl : Outport  Port=15  VectorParamsAs1DForOutWhenUnconnected=off
  Srl : Outport  Port=16  VectorParamsAs1DForOutWhenUnconnected=off
  Srr : Outport  Port=17  VectorParamsAs1DForOutWhenUnconnected=off
  Ay load transfer : Outport  Port=18
  ax load transfer : Outport  Port=19
  wires:
  Ackerman outer/1 -> "Yaw axis d,o,f "/1("Ackerman outer ")
  "Yaw axis d,o,f "/3(Yaw angle) -> Scope5/1, Yaw angle/1
  "Longtudinal axis D.O.F "/1("ax ") -> ax/1, Scope1/1
  "Longtudinal axis D.O.F "/2(X) -> X/1
  "Lateral Axis D.o.f "/1(Y) -> Scope4/1, Y/1
  "Lateral Axis D.o.f "/2(ay) -> Scope8/1, ay/1  "ay"
  "Yaw axis d,o,f "/2("yaw accelration ") -> Scope/2, "yaw accelartion "/1  "yaw acc"
  "Yaw axis d,o,f "/1("Yaw rate ") -> Scope/1, "Lateral Axis D.o.f "/10("Yaw rate "), yaw rate/1, "Slip angle and beta "/3(Yaw rate), "Slip ratio "/3(yaw rate), "Longtudinal axis D.O.F "/11("Yr ")  "yaw rate"
  "Vinput "/1 -> "Longtudinal axis D.O.F "/9(Vinput)
  "Lateral Axis D.o.f "/3(Vy) -> "Slip angle and beta "/5("Vy  "), "Slip ratio "/2(Vy), Vy/1, "Longtudinal axis D.O.F "/10("Vy "), Scope3/1  "Vy"
  "Longtudinal axis D.O.F "/3(Vx) -> "Lateral Axis D.o.f "/9(Vx), Scope2/1, "Slip ratio "/1("Vx "), Vx/1, "Slip angle and beta "/4(Vx)  "Vx"
  Fxfl/1 -> Scope6/1, "Yaw axis d,o,f "/3(Fxfl)
  "Fyfl "/1 -> "Yaw axis d,o,f "/4("Fyfl ")
  Fxfr/1 -> "Yaw axis d,o,f "/5(Fxfr), Scope6/2
  Fyfr/1 -> "Yaw axis d,o,f "/6(Fyfr)
  Fxrl/1 -> Scope7/1, "Yaw axis d,o,f "/7(Fxrl)
  Fyrl/1 -> "Yaw axis d,o,f "/8(Fyrl)
  Fxrr/1 -> Scope7/2, "Yaw axis d,o,f "/9(Fxrr)
  Fyrr/1 -> "Yaw axis d,o,f "/10(Fyrr)
  Mz fl/1 -> "Yaw axis d,o,f "/11(Mz fl)
  Mz fr/1 -> "Yaw axis d,o,f "/12(Mz fr)
  Mz rl/1 -> "Yaw axis d,o,f "/13(Mz rl)
  Mz rr/1 -> "Yaw axis d,o,f "/14(Mz rr)
  "ackerman angle "/1 -> "Longtudinal axis D.O.F "/1(ackerman outer)
  "Fxfl "/1 -> "Longtudinal axis D.O.F "/3(Fxfl)
  Fyfl/1 -> "Longtudinal axis D.O.F "/4(Fyfl)
  "Fxfr "/1 -> "Longtudinal axis D.O.F "/5(Fxfr)
  "Fyfr "/1 -> "Longtudinal axis D.O.F "/6(Fyfr)
  "Fxrr "/1 -> "Longtudinal axis D.O.F "/7(Fxrr)
  "Fxrl "/1 -> "Longtudinal axis D.O.F "/8(Fxrl)
  "Fyfl "/1 -> "Lateral Axis D.o.f "/3(Fyfl)
  "Slip ratio "/2(Sfl) -> Sfl/1  "sfl"
  "Slip ratio "/1(sfr) -> Sfr/1  "sfr"
  "Slip ratio "/3(srl) -> Srl/1  "srl"
  "Slip ratio "/4(srr) -> Srr/1  "srr"
  "Slip angle and beta "/1(alpha_fl) -> alpha_fl/1, "Slip ratio "/4(alpha_fl)  "alpha fl"
  "Slip angle and beta "/2(alpha_fr) -> alpha_fr/1, "Slip ratio "/10(alpha_fr)  "alpha fr"
  "Slip angle and beta "/3(alpha_rl) -> "Slip ratio "/5("alpha_rl "), alpha_rl/1  "alpha rl"
  "Slip angle and beta "/4(alpha_rr) -> "Slip ratio "/6(alpha_rr), alpha_rr/1  "alpha rr"
  Tb_r/1 -> "Powertrain "/1(Tb_r)
  Throtle/1 -> "Powertrain "/3(Throtle)
  Tb_f/1 -> "Powertrain "/4(Tb_ff)
  "Powertrain "/1(Wfl) -> "Slip ratio "/7("Wfl ")  "Wfl"
  "Powertrain "/2(Wrl) -> "Slip ratio "/8(Wrl)  "Wrl"
  "Powertrain "/4(Wrr) -> "Slip ratio "/9(Wrr)  "Wrr"
  Fxfl1/1 -> "Powertrain "/5("Fxfl ")
  Fxfr1/1 -> "Powertrain "/7(Fxfr)
  Fxrr1/1 -> "Powertrain "/6(Fxrr)
  Fxrl1/1 -> "Powertrain "/2(Fxrl)
  "Fxfl "/1 -> "Lateral Axis D.o.f "/5(Fxfl)
  "Fyfr "/1 -> "Lateral Axis D.o.f "/7(Fyfr)
  "Fxfr "/1 -> "Lateral Axis D.o.f "/6(Fxfr)
  "Fyrr    "/1 -> "Lateral Axis D.o.f "/4(Fyrr)
  "Fxrr "/1 -> "Lateral Axis D.o.f "/8(Fyrl)
  "Powertrain "/3(Wfr) -> "Slip ratio "/11(Wfr)  "Wfr"
  Ackerman inner/1 -> "Yaw axis d,o,f "/2("Ackerman inner ")
  "Ackerman outer "/1 -> "Slip angle and beta "/1(ackerman angle outer)
  "Ackerman inner "/1 -> "Slip angle and beta "/2("ackerman angle Inner ")
  Ackerman inner2/1 -> "Longtudinal axis D.O.F "/2(ackerman inner)
  "Ackerman inner "/1 -> "Lateral Axis D.o.f "/2("ackerman in ")
  "ackerman o "/1 -> "Lateral Axis D.o.f "/1("ackerman outer ")
  "Lateral Axis D.o.f "/4(Ay load transfer) -> Ay load transfer/1
  "Longtudinal axis D.O.F "/4(ax load transfer) -> ax load transfer/1

== system Vehicle_Model_14DOF/Subsystem/Subsystem ==
  Ff : Inport
  1/Amf : Gain  Gain=1/Amf
  Pf : Outport  VectorParamsAs1DForOutWhenUnconnected=off
  wires:
  1/Amf/1 -> Pf/1
  Ff/1 -> 1/Amf/1

== system Vehicle_Model_14DOF/Subsystem/Subsystem1 ==
  Pf : Inport
  Asf : Gain  Gain=Asf
  Fcf : Outport  VectorParamsAs1DForOutWhenUnconnected=off
  wires:
  Asf/1 -> Fcf/1
  Pf/1 -> Asf/1

== system Vehicle_Model_14DOF/Subsystem/Subsystem2 ==
  Fcf : Inport
  Gain2 : Gain  Gain=2*rb*Mb
  Tf : Outport  VectorParamsAs1DForOutWhenUnconnected=off
  wires:
  Gain2/1 -> Tf/1
  Fcf/1 -> Gain2/1

== system Vehicle_Model_14DOF/Subsystem/Subsystem3 ==
  Fr : Inport
  1/Amr : Gain  Gain=1/Amr
  Pr : Outport  VectorParamsAs1DForOutWhenUnconnected=off
  wires:
  Fr/1 -> 1/Amr/1
  1/Amr/1 -> Pr/1

== system Vehicle_Model_14DOF/Subsystem/Subsystem4 ==
  Pr : Inport
  Asr : Gain  Gain=Asr
  Fcr : Outport  VectorParamsAs1DForOutWhenUnconnected=off
  wires:
  Pr/1 -> Asr/1
  Asr/1 -> Fcr/1

== system Vehicle_Model_14DOF/Subsystem/Subsystem5 ==
  Fcr : Inport
  Gain2 : Gain  Gain=2*rb*Mb
  Tr : Outport  VectorParamsAs1DForOutWhenUnconnected=off
  wires:
  Fcr/1 -> Gain2/1
  Gain2/1 -> Tr/1

== system Vehicle_Model_14DOF/Subsystem/Subsystem6 ==
  Fb : Inport
  Gain : Gain  Gain=a/100
  Ff : Outport  VectorParamsAs1DForOutWhenUnconnected=off
  wires:
  Gain/1 -> Ff/1
  Fb/1 -> Gain/1

== system Vehicle_Model_14DOF/Subsystem/Subsystem7 ==
  Fb : Inport
  Gain : Gain  Gain=b/100
  Fr : Outport  VectorParamsAs1DForOutWhenUnconnected=off
  wires:
  Gain/1 -> Fr/1
  Fb/1 -> Gain/1

== system Vehicle_Model_14DOF/Subsystem/Subsystem8 ==
  %Fd : Inport
  Gain : Gain  Gain=(Fd*PR)
  Fb : Outport  VectorParamsAs1DForOutWhenUnconnected=off
  wires:
  Gain/1 -> Fb/1
  %Fd/1 -> Gain/1

== system Vehicle_Model_14DOF/Full vehicle 14 D.O.F /RIde1/Pitch (theta) ==
  note: You may need to change the sign of the term ( Ax * Ms * H) depending on the polarity of Ax.
  note: You may need to add an anti Pitching calculations
  Suspension Forces : Inport
  ax : Inport  Port=2
  Add : Sum
  Add1 : Sum  Inputs=--
  Add2 : Sum  Inputs=++-
  Cg to front : Gain  Gain=a
  Cg to rear : Gain  Gain=b
  Demux : Demux
  Gain : Gain  Gain=1/(Ip+((Ms+Mufl*4) * (H-Hp)^2))
  Gain1 : Gain  Gain=Ms+ (Mufl*4)
  Gain2 : Gain  Gain=Hp
  Integrator : Integrator
  Integrator1 : Integrator
  Scope : Scope
  Pitch Angle : Outport  VectorParamsAs1DForOutWhenUnconnected=off
  pitch Rate : Outport  Port=2  VectorParamsAs1DForOutWhenUnconnected=off
  wires:
  Suspension Forces/1 -> Demux/1
  Demux/1 -> Add1/1
  Demux/2 -> Add1/2
  Demux/3 -> Add/1
  Demux/4 -> Add/2
  Add1/1 -> Cg to front/1
  Add/1 -> Cg to rear/1
  Cg to front/1 -> Add2/1
  Cg to rear/1 -> Add2/2
  Add2/1 -> Gain/1
  Gain/1 -> Scope/1, Integrator/1
  Integrator/1 -> Integrator1/1, pitch Rate/1
  Integrator1/1 -> Pitch Angle/1
  ax/1 -> Gain1/1
  Gain1/1 -> Gain2/1
  Gain2/1 -> Add2/3

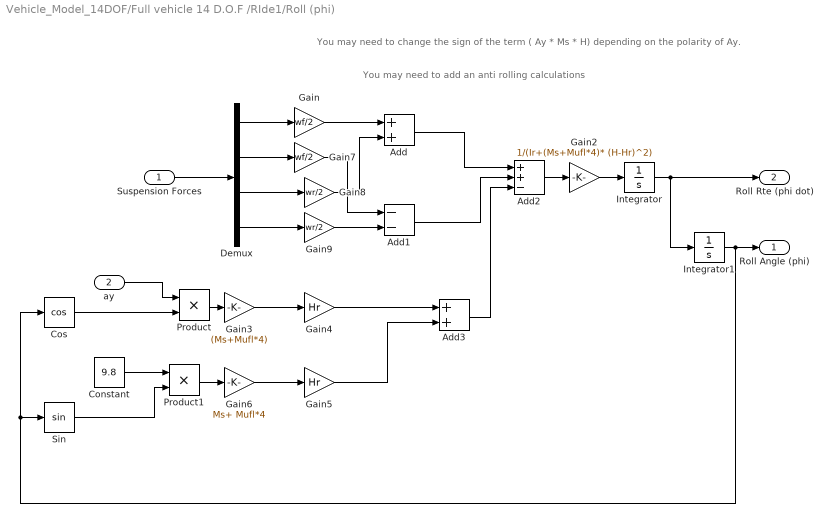
== system Vehicle_Model_14DOF/Full vehicle 14 D.O.F /RIde1/Roll (phi) ==
  note: You may need to change the sign of the term ( Ay * Ms * H) depending on the polarity of Ay.
  note: You may need to add an anti rolling calculations
  Suspension Forces : Inport
  ay : Inport  Port=2
  Add : Sum
  Add1 : Sum  Inputs=--
  Add2 : Sum  Inputs=++-
  Add3 : Sum
  Constant : Constant  Value=9.8
  Cos : Trigonometry  Operator=cos
  Demux : Demux
  Gain : Gain  Gain=wf/2
  Gain2 : Gain  Gain=1/(Ir+(Ms+Mufl*4)* (H-Hr)^2)
  Gain3 : Gain  Gain=(Ms+Mufl*4)
  Gain4 : Gain  Gain=Hr
  Gain5 : Gain  Gain=Hr
  Gain6 : Gain  Gain=Ms+ Mufl*4
  Gain7 : Gain  Gain=wf/2
  Gain8 : Gain  Gain=wr/2
  Gain9 : Gain  Gain=wr/2
  Integrator : Integrator
  Integrator1 : Integrator
  Product : Product
  Product1 : Product
  Sin : Trigonometry
  Roll Angle (phi) : Outport  VectorParamsAs1DForOutWhenUnconnected=off
  Roll Rte (phi dot) : Outport  Port=2  VectorParamsAs1DForOutWhenUnconnected=off
  wires:
  Suspension Forces/1 -> Demux/1
  Demux/3 -> Gain8/1
  Demux/2 -> Gain7/1
  Demux/1 -> Gain/1
  Demux/4 -> Gain9/1
  Add/1 -> Add2/1
  Add1/1 -> Add2/2
  Add2/1 -> Gain2/1
  Gain2/1 -> Integrator/1
  Integrator/1 -> Integrator1/1, Roll Rte (phi dot)/1
  Integrator1/1 -> Cos/1, Sin/1, Roll Angle (phi)/1
  ay/1 -> Product/1
  Gain3/1 -> Gain4/1
  Gain4/1 -> Add3/1
  Gain5/1 -> Add3/2
  Gain6/1 -> Gain5/1
  Constant/1 -> Product1/1
  Cos/1 -> Product/2
  Product/1 -> Gain3/1
  Add3/1 -> Add2/3
  Sin/1 -> Product1/2
  Product1/1 -> Gain6/1
  Gain/1 -> Add/1
  Gain7/1 -> Add1/1
  Gain9/1 -> Add1/2
  Gain8/1 -> Add/2

== system Vehicle_Model_14DOF/Full vehicle 14 D.O.F /RIde1/Sprung mass (Ms) ==
  Suspension Forces : Inport
  Add : Sum  Inputs=++++
  Demux : Demux
  Integrator : Integrator
  Integrator1 : Integrator
  car mass : Gain  Gain=1/Ms
  Zb : Outport  VectorParamsAs1DForOutWhenUnconnected=off
  Zb dot : Outport  Port=2  VectorParamsAs1DForOutWhenUnconnected=off
  Zb dot dot : Outport  Port=3  VectorParamsAs1DForOutWhenUnconnected=off
  wires:
  Suspension Forces/1 -> Demux/1
  Demux/1 -> Add/1  "Sfl"
  Demux/2 -> Add/2  "Sfr"
  Demux/3 -> Add/3  "Srl"
  Demux/4 -> Add/4  "Srr"
  Add/1 -> car mass/1
  Integrator/1 -> Integrator1/1, Zb dot/1
  car mass/1 -> Zb dot dot/1, Integrator/1
  Integrator1/1 -> Zb/1

== system Vehicle_Model_14DOF/Full vehicle 14 D.O.F /RIde1/Subsys Fz ==
  Frr : Inport
  Frl : Inport  Port=2
  vvx : Inport  Port=3
  Ffr : Inport  Port=4
  Ffl : Inport  Port=5
  Constant : Constant  Value=1/2
  Constant1 : Constant  Value=Ro
  Constant2 : Constant  Value=Cl
  Constant3 : Constant  Value=Ar
  Gain : Gain  Gain=b/(a+b)
  Gain1 : Gain  Gain=a/(a+b)
  Gain2 : Gain  Gain=1/2
  Gain3 : Gain  Gain=1/2
  Product : Product  Inputs=5
  Subsys Fzfl : Subsystem
  Subsys Fzfr : Subsystem
  Subsys Fzrl : Subsystem
  Subsys Fzrl1 : Subsystem
  Fzfl : Outport  VectorParamsAs1DForOutWhenUnconnected=off
  Fzfr : Outport  Port=2  VectorParamsAs1DForOutWhenUnconnected=off
  Fzrl : Outport  Port=3  VectorParamsAs1DForOutWhenUnconnected=off
  Fzrr : Outport  Port=4  VectorParamsAs1DForOutWhenUnconnected=off
  wires:
  Subsys Fzfl/1(Fzfl) -> Fzfl/1
  Subsys Fzfr/1(Fzfr) -> Fzfr/1
  Subsys Fzrl/1(Fzrl) -> Fzrl/1
  Subsys Fzrl1/1(Fzrr) -> Fzrr/1
  Ffl/1 -> Subsys Fzfl/1(Ffl)
  Ffr/1 -> Subsys Fzfr/1(Ffr)
  Frl/1 -> Subsys Fzrl/1(Frl)
  Frr/1 -> Subsys Fzrl1/1(Frr)
  Constant/1 -> Product/1
  Constant1/1 -> Product/2
  Constant2/1 -> Product/3
  Constant3/1 -> Product/4
  vvx/1 -> Product/5
  Product/1 -> Gain1/1, Gain/1
  Gain/1 -> Gain2/1
  Gain1/1 -> Gain3/1
  Gain2/1 -> Subsys Fzfr/2(Downforce), Subsys Fzfl/2(Downforce)  "Downforce"
  Gain3/1 -> Subsys Fzrl1/2(downforce), Subsys Fzrl/2(downforce)

== system Vehicle_Model_14DOF/Full vehicle 14 D.O.F /RIde1/Zufl ==
  Ffl : Inport
  Add : Sum  Inputs=--
  Gain : Gain  Gain=Mufl
  Gain1 : Gain  Gain=Ktfl
  Integrator : Integrator
  Integrator1 : Integrator
  Zufldot : Outport  VectorParamsAs1DForOutWhenUnconnected=off
  wires:
  Ffl/1 -> Add/2
  Gain1/1 -> Add/1
  Add/1 -> Gain/1
  Integrator/1 -> Zufldot/1, Integrator1/1
  Gain/1 -> Integrator/1
  Integrator1/1 -> Gain1/1  "zurr"

== system Vehicle_Model_14DOF/Full vehicle 14 D.O.F /RIde1/Zufr ==
  Ffr : Inport
  Add : Sum  Inputs=--
  Gain : Gain  Gain=Mufr
  Gain1 : Gain  Gain=Ktfr
  Integrator : Integrator
  Integrator1 : Integrator
  Zufr : Outport  VectorParamsAs1DForOutWhenUnconnected=off
  wires:
  Ffr/1 -> Add/2
  Gain1/1 -> Add/1
  Add/1 -> Gain/1
  Integrator/1 -> Zufr/1, Integrator1/1
  Gain/1 -> Integrator/1
  Integrator1/1 -> Gain1/1  "zurr"

== system Vehicle_Model_14DOF/Full vehicle 14 D.O.F /RIde1/Zurl ==
  Frl : Inport
  Add : Sum  Inputs=--
  Gain : Gain  Gain=Murl
  Gain1 : Gain  Gain=Ktrl
  Integrator : Integrator
  Integrator1 : Integrator
  Zurldot : Outport  VectorParamsAs1DForOutWhenUnconnected=off
  wires:
  Frl/1 -> Add/2
  Gain1/1 -> Add/1
  Add/1 -> Gain/1
  Integrator/1 -> Zurldot/1, Integrator1/1
  Gain/1 -> Integrator/1
  Integrator1/1 -> Gain1/1  "zurr"

== system Vehicle_Model_14DOF/Full vehicle 14 D.O.F /RIde1/Zurr ==
  Frr : Inport
  Add : Sum  Inputs=--
  Gain : Gain  Gain=Murr
  Gain1 : Gain  Gain=Ktrr
  Integrator : Integrator
  Integrator1 : Integrator
  Zurrdot : Outport  VectorParamsAs1DForOutWhenUnconnected=off
  wires:
  Frr/1 -> Add/2
  Add/1 -> Gain/1
  Gain/1 -> Integrator/1
  Gain1/1 -> Add/1
  Integrator/1 -> Integrator1/1, Zurrdot/1
  Integrator1/1 -> Gain1/1  "zurr"

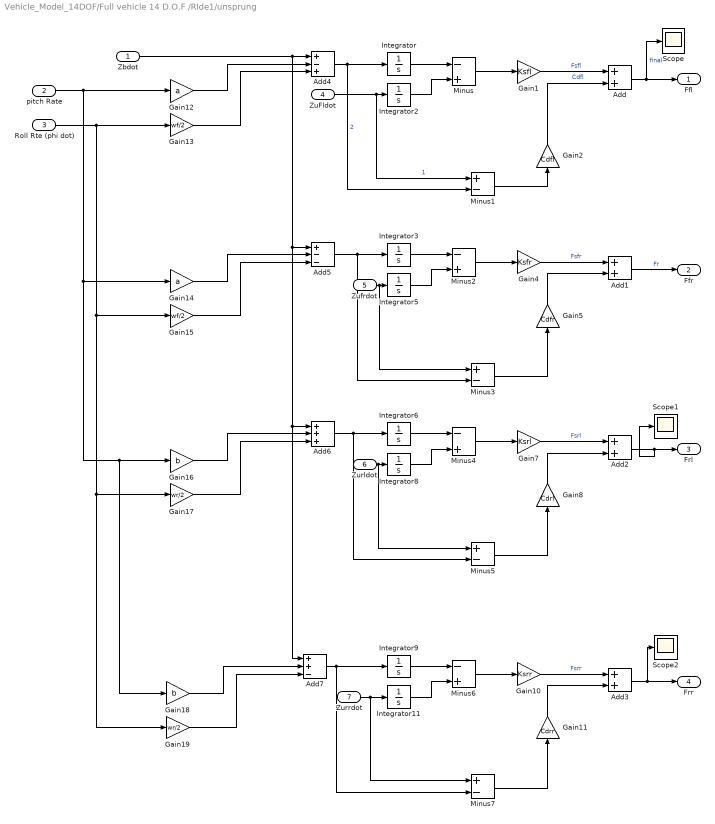
== system Vehicle_Model_14DOF/Full vehicle 14 D.O.F /RIde1/unsprung ==
  Zbdot : Inport
  pitch Rate : Inport  Port=2
  Roll Rte (phi dot) : Inport  Port=3
  ZuFldot : Inport  Port=4
  Zufrdot : Inport  Port=5
  Zurldot : Inport  Port=6
  Zurrdot : Inport  Port=7
  Add{,1..3} (4 alike) : Sum
  Add4 : Sum  Inputs=+-+
  Add5 : Sum  Inputs=+--
  Add6 : Sum  Inputs=+++
  Add7 : Sum  Inputs=++-
  Gain1 : Gain  Gain=Ksfl
  Gain10 : Gain  Gain=Ksrr
  Gain11 : Gain  Gain=Cdrr
  Gain12 : Gain  Gain=a
  Gain13 : Gain  Gain=wf/2
  Gain14 : Gain  Gain=a
  Gain15 : Gain  Gain=wf/2
  Gain16 : Gain  Gain=b
  Gain17 : Gain  Gain=wr/2
  Gain18 : Gain  Gain=b
  Gain19 : Gain  Gain=wr/2
  Gain2 : Gain  Gain=Cdfl
  Gain4 : Gain  Gain=Ksfr
  Gain5 : Gain  Gain=Cdfr
  Gain7 : Gain  Gain=Ksrl
  Gain8 : Gain  Gain=Cdrl
  Integrator{,2..3,5..6,8..9,11} (8 alike) : Integrator
  Minus{,2,4,6} (4 alike) : Sum  Inputs=-+
  Minus{1,3,5,7} (4 alike) : Sum  Inputs=+-
  Scope : Scope
  Scope1 : Scope
  Scope2 : Scope
  Ffl : Outport  VectorParamsAs1DForOutWhenUnconnected=off
  Ffr : Outport  Port=2  VectorParamsAs1DForOutWhenUnconnected=off
  Frl : Outport  Port=3  VectorParamsAs1DForOutWhenUnconnected=off
  Frr : Outport  Port=4  VectorParamsAs1DForOutWhenUnconnected=off
  wires:
  Integrator/1 -> Minus/1
  Minus/1 -> Gain1/1
  Gain1/1 -> Add/1  "Fsfl"
  Gain2/1 -> Add/2  "Cdfl"
  Add/1 -> Scope/1, Ffl/1  "final"
  Integrator2/1 -> Minus/2
  Gain5/1 -> Add1/2
  Minus2/1 -> Gain4/1
  Integrator5/1 -> Minus2/2
  Add1/1 -> Ffr/1  "Fr"
  Gain4/1 -> Add1/1  "Fsfr"
  Integrator3/1 -> Minus2/1
  Gain8/1 -> Add2/2
  Minus4/1 -> Gain7/1
  Integrator8/1 -> Minus4/2
  Add2/1 -> Scope1/1, Frl/1
  Gain7/1 -> Add2/1  "Fsrl"
  Integrator6/1 -> Minus4/1
  Gain11/1 -> Add3/2
  Minus6/1 -> Gain10/1
  Integrator11/1 -> Minus6/2
  Add3/1 -> Scope2/1, Frr/1
  Gain10/1 -> Add3/1  "Fsrr"
  Zbdot/1 -> Add7/1, Add6/1, Add5/1, Add4/1
  Integrator9/1 -> Minus6/1
  Add4/1 -> Integrator/1, Minus1/2  "2"
  Gain12/1 -> Add4/2
  Gain13/1 -> Add4/3
  Add5/1 -> Integrator3/1, Minus3/2
  Gain14/1 -> Add5/2
  Gain15/1 -> Add5/3
  Add6/1 -> Minus5/2, Integrator6/1
  Gain16/1 -> Add6/2
  Gain17/1 -> Add6/3
  Add7/1 -> Minus7/2, Integrator9/1
  pitch Rate/1 -> Gain12/1, Gain18/1, Gain16/1, Gain14/1
  Roll Rte (phi dot)/1 -> Gain15/1, Gain17/1, Gain19/1, Gain13/1
  Gain19/1 -> Add7/3
  Gain18/1 -> Add7/2
  ZuFldot/1 -> Minus1/1, Integrator2/1  "1"
  Zufrdot/1 -> Minus3/1, Integrator5/1
  Zurldot/1 -> Minus5/1, Integrator8/1
  Zurrdot/1 -> Minus7/1, Integrator11/1
  Minus1/1 -> Gain2/1
  Minus3/1 -> Gain5/1
  Minus5/1 -> Gain8/1
  Minus7/1 -> Gain11/1

== system Vehicle_Model_14DOF/Full vehicle 14 D.O.F /Tiremodel/LCO width 6 psi 10 ==
  Fz : Inport
  S : Inport  Port=2
  alpha : Inport  Port=3
  Fx : Subsystem
  Fz1 : InportShadow
  Fz2 : InportShadow
  In1 : InportShadow  Port=3
  fy : Subsystem
  fy1 : Subsystem
  "Fx  " : Outport  VectorParamsAs1DForOutWhenUnconnected=off
  Fy : Outport  Port=2  VectorParamsAs1DForOutWhenUnconnected=off
  Mz : Outport  Port=3  VectorParamsAs1DForOutWhenUnconnected=off
  wires:
  Fz/1 -> Fx/1(Fz)
  In1/1 -> fy1/2(alpha)
  Fz2/1 -> fy1/1(Fz1)
  Fz1/1 -> fy/1(Fz)
  alpha/1 -> fy/2(Slip angle)
  fy/1("Fy  ") -> Fy/1
  fy1/1(mmz) -> Mz/1
  Fx/1("Fx  ") -> "Fx  "/1
  S/1 -> Fx/2(In3)

== system Vehicle_Model_14DOF/Full vehicle 14 D.O.F /Tiremodel/LCO width 6 psi 14 ==
  Fz : Inport
  S : Inport  Port=2
  alpha : Inport  Port=3
  Fx : Subsystem
  Fz1 : InportShadow
  Fz2 : InportShadow
  In1 : InportShadow  Port=3
  fy : Subsystem
  fy1 : Subsystem
  "Fx  " : Outport  VectorParamsAs1DForOutWhenUnconnected=off
  Fy : Outport  Port=2  VectorParamsAs1DForOutWhenUnconnected=off
  Mz : Outport  Port=3  VectorParamsAs1DForOutWhenUnconnected=off
  wires:
  Fz/1 -> Fx/1(Fz)
  In1/1 -> fy1/2(alpha)
  Fz2/1 -> fy1/1(Fz1)
  Fz1/1 -> fy/1(Fz)
  alpha/1 -> fy/2(Slip angle)
  fy/1("Fy  ") -> Fy/1
  fy1/1(mmz) -> Mz/1
  Fx/1("Fx  ") -> "Fx  "/1
  S/1 -> Fx/2(In3)

== system Vehicle_Model_14DOF/Full vehicle 14 D.O.F /Tiremodel/R25b width 6 psi 10 ==
  Fz : Inport
  S : Inport  Port=2
  alpha : Inport  Port=3
  Fx : Subsystem
  Fz1 : InportShadow
  Fz2 : InportShadow
  In1 : InportShadow  Port=3
  fy : Subsystem
  fy1 : Subsystem
  "Fx  " : Outport  VectorParamsAs1DForOutWhenUnconnected=off
  Fy : Outport  Port=2  VectorParamsAs1DForOutWhenUnconnected=off
  Mz : Outport  Port=3  VectorParamsAs1DForOutWhenUnconnected=off
  wires:
  Fz/1 -> Fx/1(Fz)
  In1/1 -> fy1/2(alpha)
  Fz2/1 -> fy1/1(Fz1)
  Fz1/1 -> fy/1(Fz)
  alpha/1 -> fy/2(Slip angle)
  fy/1("Fy  ") -> Fy/1
  fy1/1(mmz) -> Mz/1
  Fx/1("Fx  ") -> "Fx  "/1
  S/1 -> Fx/2(In3)

== system Vehicle_Model_14DOF/Full vehicle 14 D.O.F /Tiremodel/R25b width 6 psi 14 ==
  Fz : Inport
  S : Inport  Port=2
  alpha : Inport  Port=3
  Fx : Subsystem
  Fz1 : InportShadow
  Fz2 : InportShadow
  In1 : InportShadow  Port=3
  fy : Subsystem
  fy1 : Subsystem
  "Fx  " : Outport  VectorParamsAs1DForOutWhenUnconnected=off
  Fy : Outport  Port=2  VectorParamsAs1DForOutWhenUnconnected=off
  Mz : Outport  Port=3  VectorParamsAs1DForOutWhenUnconnected=off
  wires:
  Fz/1 -> Fx/1(Fz)
  In1/1 -> fy1/2(alpha)
  Fz2/1 -> fy1/1(Fz1)
  Fz1/1 -> fy/1(Fz)
  alpha/1 -> fy/2(Slip angle)
  fy/1("Fy  ") -> Fy/1
  fy1/1(mmz) -> Mz/1
  Fx/1("Fx  ") -> "Fx  "/1
  S/1 -> Fx/2(In3)

== system Vehicle_Model_14DOF/Full vehicle 14 D.O.F /Tiremodel/R25b width 7 psi 10 ==
  Fz : Inport
  S : Inport  Port=2
  alpha : Inport  Port=3
  Fx : Subsystem
  Fz1 : InportShadow
  Fz2 : InportShadow
  In1 : InportShadow  Port=3
  MZ : Subsystem
  fy : Subsystem
  "Fx  " : Outport  VectorParamsAs1DForOutWhenUnconnected=off
  Fy : Outport  Port=2  VectorParamsAs1DForOutWhenUnconnected=off
  Mz : Outport  Port=3  VectorParamsAs1DForOutWhenUnconnected=off
  wires:
  Fz/1 -> Fx/1(Fz)
  In1/1 -> MZ/2(alpha)
  Fz2/1 -> MZ/1(Fz1)
  Fz1/1 -> fy/1(Fz)
  alpha/1 -> fy/2(Slip angle)
  fy/1("Fy  ") -> Fy/1
  MZ/1(mmz) -> Mz/1
  Fx/1("Fx  ") -> "Fx  "/1
  S/1 -> Fx/2(In3)

== system Vehicle_Model_14DOF/Full vehicle 14 D.O.F /Tiremodel/R25b width 7 psi 14 ==
  Fz : Inport
  S : Inport  Port=2
  alpha : Inport  Port=3
  Fx : Subsystem
  Fz1 : InportShadow
  Fz2 : InportShadow
  In1 : InportShadow  Port=3
  fy : Subsystem
  fy1 : Subsystem
  "Fx  " : Outport  VectorParamsAs1DForOutWhenUnconnected=off
  Fy : Outport  Port=2  VectorParamsAs1DForOutWhenUnconnected=off
  Mz : Outport  Port=3  VectorParamsAs1DForOutWhenUnconnected=off
  wires:
  Fz/1 -> Fx/1(Fz)
  In1/1 -> fy1/2(alpha)
  Fz2/1 -> fy1/1(Fz1)
  Fz1/1 -> fy/1(Fz)
  alpha/1 -> fy/2(Slip angle)
  fy/1("Fy  ") -> Fy/1
  fy1/1(mmz) -> Mz/1
  Fx/1("Fx  ") -> "Fx  "/1
  S/1 -> Fx/2(In3)

== system Vehicle_Model_14DOF/Full vehicle 14 D.O.F /Tiremodel/Tire front left ==
  Fz : Inport
  S : Inport  Port=2
  alpha : Inport  Port=3
  Fx : Subsystem
  Fz1 : InportShadow
  Fz2 : InportShadow
  In1 : InportShadow  Port=3
  fy : Subsystem
  fy1 : Subsystem
  "Fx  " : Outport  VectorParamsAs1DForOutWhenUnconnected=off
  Fy : Outport  Port=2  VectorParamsAs1DForOutWhenUnconnected=off
  Mz : Outport  Port=3  VectorParamsAs1DForOutWhenUnconnected=off
  wires:
  Fz/1 -> Fx/1(Fz)
  In1/1 -> fy1/2(alpha)
  Fz2/1 -> fy1/1(Fz1)
  Fz1/1 -> fy/1(Fz)
  alpha/1 -> fy/2(Slip angle)
  fy/1("Fy  ") -> Fy/1
  fy1/1(mmz) -> Mz/1
  Fx/1("Fx  ") -> "Fx  "/1
  S/1 -> Fx/2(S)

== system Vehicle_Model_14DOF/Full vehicle 14 D.O.F /Tiremodel/Tire front right ==
  Fz : Inport
  S : Inport  Port=2
  alpha : Inport  Port=3
  Fx : Subsystem
  Fz1 : InportShadow
  Fz2 : InportShadow
  In1 : InportShadow  Port=3
  fy : Subsystem
  fy1 : Subsystem
  "Fx  " : Outport  VectorParamsAs1DForOutWhenUnconnected=off
  Fy : Outport  Port=2  VectorParamsAs1DForOutWhenUnconnected=off
  Mz : Outport  Port=3  VectorParamsAs1DForOutWhenUnconnected=off
  wires:
  S/1 -> Fx/2(In3)
  Fx/1("Fx  ") -> "Fx  "/1
  fy1/1(mmz) -> Mz/1
  fy/1("Fy  ") -> Fy/1
  alpha/1 -> fy/2(Slip angle)
  Fz1/1 -> fy/1(Fz)
  Fz2/1 -> fy1/1(Fz1)
  In1/1 -> fy1/2(alpha)
  Fz/1 -> Fx/1(Fz)

== system Vehicle_Model_14DOF/Full vehicle 14 D.O.F /Tiremodel/Tire rear Right ==
  Fz : Inport
  S : Inport  Port=2
  alpha : Inport  Port=3
  Fx : Subsystem
  Fz1 : InportShadow
  Fz2 : InportShadow
  In1 : InportShadow  Port=3
  fy : Subsystem
  fy1 : Subsystem
  "Fx  " : Outport  VectorParamsAs1DForOutWhenUnconnected=off
  Fy : Outport  Port=2  VectorParamsAs1DForOutWhenUnconnected=off
  Mz : Outport  Port=3  VectorParamsAs1DForOutWhenUnconnected=off
  wires:
  Fz/1 -> Fx/1(Fz)
  In1/1 -> fy1/2(alpha)
  Fz2/1 -> fy1/1(Fz1)
  Fz1/1 -> fy/1(Fz)
  alpha/1 -> fy/2(Slip angle)
  fy/1("Fy  ") -> Fy/1
  fy1/1(mmz) -> Mz/1
  Fx/1("Fx  ") -> "Fx  "/1
  S/1 -> Fx/2(In3)

== system Vehicle_Model_14DOF/Full vehicle 14 D.O.F /Tiremodel/Tire rear left ==
  Fz : Inport
  S : Inport  Port=2
  alpha : Inport  Port=3
  Fx : Subsystem
  Fz1 : InportShadow
  Fz2 : InportShadow
  In1 : InportShadow  Port=3
  fy : Subsystem
  fy1 : Subsystem
  "Fx  " : Outport  VectorParamsAs1DForOutWhenUnconnected=off
  Fy : Outport  Port=2  VectorParamsAs1DForOutWhenUnconnected=off
  Mz : Outport  Port=3  VectorParamsAs1DForOutWhenUnconnected=off
  wires:
  S/1 -> Fx/2(In3)
  Fx/1("Fx  ") -> "Fx  "/1
  fy1/1(mmz) -> Mz/1
  fy/1("Fy  ") -> Fy/1
  alpha/1 -> fy/2(Slip angle)
  Fz1/1 -> fy/1(Fz)
  Fz2/1 -> fy1/1(Fz1)
  In1/1 -> fy1/2(alpha)
  Fz/1 -> Fx/1(Fz)
